simulink model "BAS_MPC_TV"  (R2018b)
settings: Solver=VariableStepAuto  StartTime=0.0  StopTime=10.0  RelTol=1e-3
values from neighbouring files (symbols this model uses):
  a = 1    [adaptive_mpc_tv.mat]
  b = 0.5    [adaptive_mpc_tv.mat]
  Izz = 100    [adaptive_mpc_tv.mat]
  M = 300    [adaptive_mpc_tv.mat]
  Rt = 0.226    [adaptive_mpc_tv.mat]
  track = 1.2    [adaptive_mpc_tv.mat]
  Ts = 0.02    [adaptive_mpc_tv.mat]
(part 1 of 2)
settings Model: Creator=littune  LastModifiedBy=littune

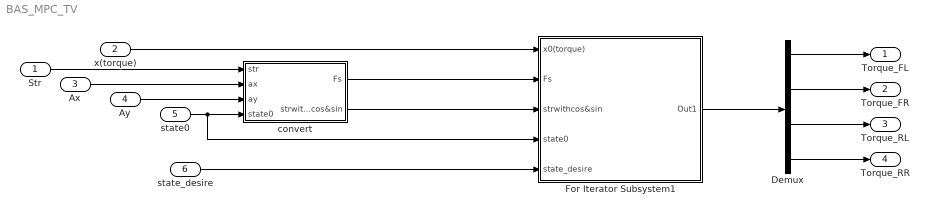
== system BAS_MPC_TV ==
  Str : Inport
  x(torque) : Inport  Port=2
  Ax : Inport  Port=3
  Ay : Inport  Port=4
  state0 : Inport  Port=5
  state_desire : Inport  Port=6
  Demux : Demux
  For Iterator Subsystem1 : Subsystem  TreatAsAtomicUnit=on
  convert : Subsystem
  Torque_FL : Outport
  Torque_FR : Outport  Port=2
  Torque_RL : Outport  Port=3
  Torque_RR : Outport  Port=4
  wires:
  convert/1(Fs) -> For Iterator Subsystem1/2(Fs)
  convert/2(strwithcos&sin) -> For Iterator Subsystem1/3(strwithcos&sin)
  Str/1 -> convert/1(str)
  x(torque)/1 -> For Iterator Subsystem1/1(x0(torque))
  Ax/1 -> convert/2(ax)
  Ay/1 -> convert/3(ay)
  state0/1 -> For Iterator Subsystem1/4(state0), convert/4(state0)
  state_desire/1 -> For Iterator Subsystem1/5(state_desire)
  For Iterator Subsystem1/1(Out1) -> Demux/1
  Demux/1 -> Torque_FL/1
  Demux/2 -> Torque_FR/1
  Demux/3 -> Torque_RL/1
  Demux/4 -> Torque_RR/1

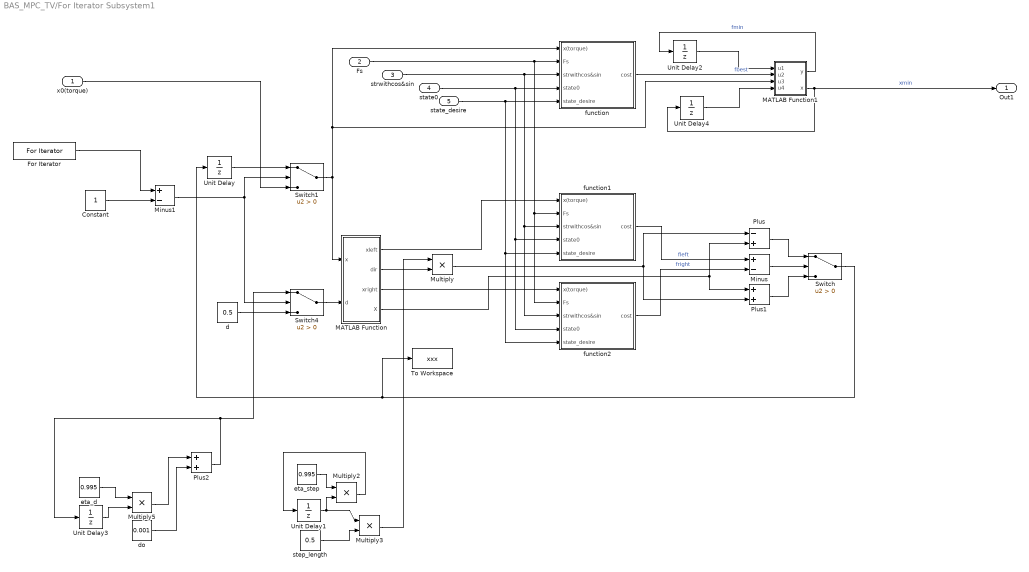
== system BAS_MPC_TV/For Iterator Subsystem1 ==
  x0(torque) : Inport
  Fs : Inport  Port=2
  strwithcos&sin : Inport  Port=3
  state0 : Inport  Port=4
  state_desire : Inport  Port=5
  Constant : Constant
  For Iterator : ForIterator  ResetStates=reset  IterationLimit=200
  MATLAB Function : MATLAB Function  TreatAsAtomicUnit=on
  MATLAB Function1 : MATLAB Function  TreatAsAtomicUnit=on
  Minus : Sum  Inputs=+-
  Minus1 : Sum  Inputs=+-
  Multiply{,2..3,5} (4 alike) : Product
  Plus : Sum  Inputs=-+
  Plus1 : Sum
  Plus2 : Sum
  Switch : Switch  Criteria=u2 > Threshold
  Switch1 : Switch  Criteria=u2 > Threshold
  Switch4 : Switch  Criteria=u2 > Threshold
  To Workspace : ToWorkspace  VariableName=xxx  SaveFormat=Timeseries  SampleTime=-1
  Unit Delay : UnitDelay  SampleTime=-1
  Unit Delay1 : UnitDelay  InitialCondition=1  SampleTime=-1
  Unit Delay2 : UnitDelay  InitialCondition=inf  SampleTime=-1
  Unit Delay3 : UnitDelay  InitialCondition=0.5  SampleTime=-1
  Unit Delay4 : UnitDelay  SampleTime=-1
  d : Constant  Value=0.5
  do : Constant  Value=0.001
  eta_d : Constant  Value=0.995
  eta_step : Constant  Value=0.995
  function : Subsystem
  function1 : Subsystem
  function2 : Subsystem
  step_length : Constant  Value=0.5
  Out1 : Outport
  wires:
  MATLAB Function/1(xleft) -> function1/1(x(torque))
  function/1(cost) -> MATLAB Function1/2(u2)  "fbest"
  strwithcos&sin/1 -> function/3(strwithcos&sin), function2/3(strwithcos&sin), function1/3(strwithcos&sin)
  MATLAB Function/3(xright) -> function2/1(x(torque))
  state0/1 -> function/4(state0), function2/4(state0), function1/4(state0)
  state_desire/1 -> function/5(state_desire), function2/5(state_desire), function1/5(state_desire)
  Fs/1 -> function/2(Fs), function2/2(Fs), function1/2(Fs)
  function1/1(cost) -> Minus/1  "fleft"
  function2/1(cost) -> Minus/2  "fright"
  Minus/1 -> Switch/2
  MATLAB Function/2(dir) -> Multiply/2
  Multiply/1 -> Plus/1, Plus1/2
  MATLAB Function/4(X) -> Plus1/1, Plus/2
  Plus/1 -> Switch/1
  Plus1/1 -> Switch/3
  Switch/1 -> Unit Delay/1, To Workspace/1
  Unit Delay/1 -> Switch1/1
  Switch1/1 -> MATLAB Function/1(x), function/1(x(torque)), MATLAB Function1/3(u3)
  Constant/1 -> Minus1/2
  Minus1/1 -> Switch4/2, Switch1/2
  eta_step/1 -> Multiply2/1
  Multiply2/1 -> Unit Delay1/1
  Unit Delay1/1 -> Multiply3/1, Multiply2/2
  step_length/1 -> Multiply3/2
  Multiply3/1 -> Multiply/1
  For Iterator/1 -> Minus1/1
  Multiply5/1 -> Plus2/1
  do/1 -> Plus2/2
  Switch4/1 -> MATLAB Function/2(d)
  d/1 -> Switch4/3
  Plus2/1 -> Switch4/1, Unit Delay3/1
  Unit Delay3/1 -> Multiply5/2
  eta_d/1 -> Multiply5/1
  x0(torque)/1 -> Switch1/3
  Unit Delay2/1 -> MATLAB Function1/1(u1)
  MATLAB Function1/1(y) -> Unit Delay2/1  "fmin"
  Unit Delay4/1 -> MATLAB Function1/4(u4)
  MATLAB Function1/2(x) -> Unit Delay4/1, Out1/1  "xmin"

== system BAS_MPC_TV/convert ==
  str : Inport
  ax : Inport  Port=2
  ay : Inport  Port=3
  state0 : Inport  Port=4
  Cos : Trigonometry  Operator=cos
  Cos1 : Trigonometry  Operator=cos
  Demux : Demux  Outputs=3
  MATLAB Function : MATLAB Function  TreatAsAtomicUnit=on
  MATLAB Function1 : MATLAB Function  TreatAsAtomicUnit=on
  Multiply{,1..3} (4 alike) : Product
  Mux : Mux
  Mux1 : Mux  Inputs=5
  Sin : Trigonometry
  Sin1 : Trigonometry
  ratio : Gain  Gain=1/5
  Fs : Outport
  strwithcos&sin : Outport  Port=2
  wires:
  ratio/1 -> Cos/1, Sin/1, Cos1/1, Mux1/5, Sin1/1
  str/1 -> ratio/1
  MATLAB Function/2(Fzfr) -> Multiply1/1
  ax/1 -> MATLAB Function/1(ax)
  ay/1 -> MATLAB Function/2(ay)
  Mux/1 -> Fs/1  "Fs"
  Mux1/1 -> strwithcos&sin/1  "strwithcos&sin"
  MATLAB Function1/4(usrr) -> Multiply3/2
  Sin/1 -> Mux1/1
  Multiply2/1 -> Mux/3  "Fs_RL"
  Multiply3/1 -> Mux/4  "Fs_RR"
  Multiply1/1 -> Mux/2  "Fs_FR"
  Multiply/1 -> Mux/1  "Fs_FL"
  MATLAB Function/4(Fzrr) -> Multiply3/1
  MATLAB Function/3(Fzrl) -> Multiply2/1
  Cos/1 -> Mux1/2
  Demux/2 -> MATLAB Function1/2(Vy0)
  state0/1 -> Demux/1
  MATLAB Function1/2(usfr) -> Multiply1/2
  Demux/3 -> MATLAB Function1/3(yawrate0)
  MATLAB Function1/3(usrl) -> Multiply2/2
  Cos1/1 -> Mux1/4
  Sin1/1 -> Mux1/3
  MATLAB Function1/1(usfl) -> Multiply/2
  Demux/1 -> MATLAB Function1/1(Vx0)
  MATLAB Function/1(Fzfl) -> Multiply/1

== system BAS_MPC_TV/For Iterator Subsystem1/function ==
  x(torque) : Inport
  Fs : Inport  Port=2
  strwithcos&sin : Inport  Port=3
  state0 : Inport  Port=4
  state_desire : Inport  Port=5
  10layer_model : Subsystem
  Gain : Gain  Gain=1/Rt
  Limitation : Subsystem
  SumFx : Subsystem
  SumFx1 : Subsystem
  cost : Outport
  wires:
  Gain/1 -> SumFx1/3(Ft), SumFx/3(Ft)
  state_desire/1 -> 10layer_model/4(state_desire)
  state0/1 -> 10layer_model/3(state0)
  strwithcos&sin/1 -> SumFx1/1(Strwithcos&sin), SumFx/1(Strwithcos&sin)
  x(torque)/1 -> Gain/1
  SumFx/1(Fx) -> 10layer_model/1(Fx)
  SumFx1/1(Fy) -> 10layer_model/2(Fy)
  Fs/1 -> SumFx/2(Fs), SumFx1/2(Fs)
  10layer_model/1(Fun) -> cost/1

== system BAS_MPC_TV/For Iterator Subsystem1/function1 ==
  x(torque) : Inport
  Fs : Inport  Port=2
  strwithcos&sin : Inport  Port=3
  state0 : Inport  Port=4
  state_desire : Inport  Port=5
  10layer_model : Subsystem
  Gain : Gain  Gain=1/Rt
  SumFx : Subsystem
  SumFx1 : Subsystem
  cost : Outport
  wires:
  Gain/1 -> SumFx1/3(Ft), SumFx/3(Ft)
  state_desire/1 -> 10layer_model/4(state_desire)
  state0/1 -> 10layer_model/3(state0)
  strwithcos&sin/1 -> SumFx1/1(Strwithcos&sin), SumFx/1(Strwithcos&sin)
  x(torque)/1 -> Gain/1
  SumFx/1(Fx) -> 10layer_model/1(Fx)
  SumFx1/1(Fy) -> 10layer_model/2(Fy)
  Fs/1 -> SumFx/2(Fs), SumFx1/2(Fs)
  10layer_model/1(Fun) -> cost/1

== system BAS_MPC_TV/For Iterator Subsystem1/function2 ==
  x(torque) : Inport
  Fs : Inport  Port=2
  strwithcos&sin : Inport  Port=3
  state0 : Inport  Port=4
  state_desire : Inport  Port=5
  10layer_model : Subsystem
  Gain : Gain  Gain=1/Rt
  SumFx : Subsystem
  SumFx1 : Subsystem
  cost : Outport
  wires:
  Gain/1 -> SumFx1/3(Ft), SumFx/3(Ft)
  state_desire/1 -> 10layer_model/4(state_desire)
  state0/1 -> 10layer_model/3(state0)
  strwithcos&sin/1 -> SumFx1/1(Strwithcos&sin), SumFx/1(Strwithcos&sin)
  x(torque)/1 -> Gain/1
  SumFx/1(Fx) -> 10layer_model/1(Fx)
  SumFx1/1(Fy) -> 10layer_model/2(Fy)
  Fs/1 -> SumFx/2(Fs), SumFx1/2(Fs)
  10layer_model/1(Fun) -> cost/1

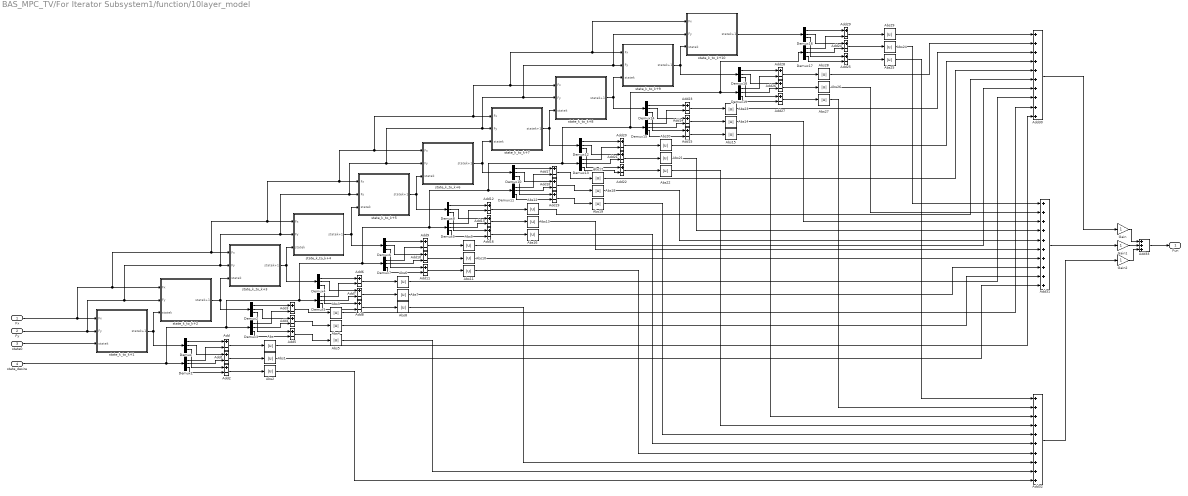
== system BAS_MPC_TV/For Iterator Subsystem1/function/10layer_model ==
  Fx : Inport
  Fy : Inport  Port=2
  state0 : Inport  Port=3
  state_desire : Inport  Port=4
  Abs{,1..29} (30 alike) : Abs
  Add{,1..29} (30 alike) : Sum  Inputs=+-
  Add30 : Sum  Inputs=10
  Add31 : Sum  Inputs=10
  Add32 : Sum  Inputs=10
  Add33 : Sum  Inputs=3
  Demux{,1..19} (20 alike) : Demux  Outputs=3
  Gain : Gain
  Gain1 : Gain
  Gain2 : Gain
  state_k_to_k+1 : Subsystem
  state_k_to_k+10 : Subsystem
  state_k_to_k+2 : Subsystem
  state_k_to_k+3 : Subsystem
  state_k_to_k+4 : Subsystem
  state_k_to_k+5 : Subsystem
  state_k_to_k+6 : Subsystem
  state_k_to_k+7 : Subsystem
  state_k_to_k+8 : Subsystem
  state_k_to_k+9 : Subsystem
  Fun : Outport
  wires:
  state_k_to_k+1/1(statek+1) -> state_k_to_k+2/3(statek), Demux/1
  state0/1 -> state_k_to_k+1/3(statek)
  Fx/1 -> state_k_to_k+10/1(Fx), state_k_to_k+9/1(Fx), state_k_to_k+8/1(Fx), state_k_to_k+7/1(Fx), state_k_to_k+6/1(Fx), state_k_to_k+5/1(Fx), state_k_to_k+4/1(Fx), state_k_to_k+3/1(Fx), state_k_to_k+2/1(Fx), state_k_to_k+1/1(Fx)
  Fy/1 -> state_k_to_k+10/2(Fy), state_k_to_k+9/2(Fy), state_k_to_k+8/2(Fy), state_k_to_k+7/2(Fy), state_k_to_k+6/2(Fy), state_k_to_k+5/2(Fy), state_k_to_k+4/2(Fy), state_k_to_k+3/2(Fy), state_k_to_k+2/2(Fy), state_k_to_k+1/2(Fy)
  Demux/1 -> Add/1
  Demux1/1 -> Add/2
  Demux/2 -> Add1/1
  Demux1/2 -> Add1/2
  Demux/3 -> Add2/1
  Demux1/3 -> Add2/2
  Add/1 -> Abs/1
  Add1/1 -> Abs1/1
  Add2/1 -> Abs2/1
  Demux2/1 -> Add3/1
  Demux2/3 -> Add5/1
  Demux3/3 -> Add5/2
  Demux2/2 -> Add4/1
  Demux3/1 -> Add3/2
  Add4/1 -> Abs4/1
  Add3/1 -> Abs3/1
  Add5/1 -> Abs5/1
  state_k_to_k+2/1(statek+1) -> Demux2/1, state_k_to_k+3/3(statek)
  Demux3/2 -> Add4/2
  Demux4/1 -> Add6/1
  Demux4/3 -> Add8/1
  Demux5/3 -> Add8/2
  Demux5/2 -> Add7/2
  Add11/1 -> Abs11/1
  Demux7/2 -> Add10/2
  Demux6/2 -> Add10/1
  Demux7/3 -> Add11/2
  Demux4/2 -> Add7/1
  Demux5/1 -> Add6/2
  Add10/1 -> Abs10/1
  Add9/1 -> Abs9/1
  Demux7/1 -> Add9/2
  Add6/1 -> Abs6/1
  Add8/1 -> Abs8/1
  Demux6/1 -> Add9/1
  Demux6/3 -> Add11/1
  Add7/1 -> Abs7/1
  state_k_to_k+4/1(statek+1) -> Demux6/1, state_k_to_k+5/3(statek)
  state_k_to_k+3/1(statek+1) -> Demux4/1, state_k_to_k+4/3(statek)
  state_k_to_k+7/1(statek+1) -> Demux12/1, state_k_to_k+8/3(statek)
  state_k_to_k+8/1(statek+1) -> Demux14/1, state_k_to_k+9/3(statek)
  Demux8/1 -> Add12/1
  Demux8/3 -> Add16/1
  Demux9/3 -> Add16/2
  Demux9/2 -> Add13/2
  Add19/1 -> Abs19/1
  Demux11/2 -> Add18/2
  Demux10/2 -> Add18/1
  Demux11/3 -> Add19/2
  Demux8/2 -> Add13/1
  Demux9/1 -> Add12/2
  Add18/1 -> Abs18/1
  Demux10/1 -> Add17/1
  Demux10/3 -> Add19/1
  Add12/1 -> Abs12/1
  Add21/1 -> Abs21/1
  Demux14/3 -> Add15/1
  Add16/1 -> Abs16/1
  Add20/1 -> Abs20/1
  Add17/1 -> Abs17/1
  Add22/1 -> Abs22/1
  Add23/1 -> Abs23/1
  Demux15/1 -> Add23/2
  Add14/1 -> Abs14/1
  Demux13/1 -> Add20/2
  Demux15/3 -> Add15/2
  Demux12/2 -> Add21/1
  Demux15/2 -> Add14/2
  Add15/1 -> Abs15/1
  Demux14/1 -> Add23/1
  Demux13/3 -> Add22/2
  Demux12/3 -> Add22/1
  Demux11/1 -> Add17/2
  Demux13/2 -> Add21/2
  Demux14/2 -> Add14/1
  Add13/1 -> Abs13/1
  state_k_to_k+6/1(statek+1) -> Demux10/1, state_k_to_k+7/3(statek)
  state_k_to_k+5/1(statek+1) -> Demux8/1, state_k_to_k+6/3(statek)
  Demux12/1 -> Add20/1
  Demux16/2 -> Add24/1
  state_k_to_k+10/1(statek+1) -> Demux16/1
  Add25/1 -> Abs25/1
  Demux17/3 -> Add25/2
  Add24/1 -> Abs24/1
  Demux16/1 -> Add29/1
  Demux17/2 -> Add24/2
  Demux16/3 -> Add25/1
  Demux17/1 -> Add29/2
  Add29/1 -> Abs29/1
  state_desire/1 -> Demux17/1, Demux19/1, Demux15/1, Demux13/1, Demux11/1, Demux9/1, Demux7/1, Demux5/1, Demux3/1, Demux1/1
  Add28/1 -> Abs28/1
  Demux19/2 -> Add26/2
  Demux19/1 -> Add28/2
  Demux18/1 -> Add28/1
  Demux18/3 -> Add27/1
  state_k_to_k+9/1(statek+1) -> Demux18/1, state_k_to_k+10/3(statek)
  Demux19/3 -> Add27/2
  Add27/1 -> Abs27/1
  Add26/1 -> Abs26/1
  Demux18/2 -> Add26/1
  Abs29/1 -> Add30/1
  Abs28/1 -> Add30/2
  Abs23/1 -> Add30/3
  Abs20/1 -> Add30/4
  Abs17/1 -> Add30/5
  Abs12/1 -> Add30/6
  Abs9/1 -> Add30/7
  Abs6/1 -> Add30/8
  Abs3/1 -> Add30/9
  Abs/1 -> Add30/10
  Add30/1 -> Gain/1
  Add31/1 -> Gain1/1
  Abs4/1 -> Add31/9
  Abs10/1 -> Add31/7
  Abs7/1 -> Add31/8
  Abs14/1 -> Add31/3
  Abs18/1 -> Add31/5
  Abs1/1 -> Add31/10
  Abs26/1 -> Add31/2
  Abs24/1 -> Add31/1
  Abs13/1 -> Add31/6
  Abs21/1 -> Add31/4
  Add32/1 -> Gain2/1
  Abs5/1 -> Add32/9
  Abs11/1 -> Add32/7
  Abs8/1 -> Add32/8
  Abs15/1 -> Add32/3
  Abs19/1 -> Add32/5
  Abs2/1 -> Add32/10
  Abs27/1 -> Add32/2
  Abs25/1 -> Add32/1
  Abs16/1 -> Add32/6
  Abs22/1 -> Add32/4
  Gain/1 -> Add33/1
  Gain1/1 -> Add33/2
  Gain2/1 -> Add33/3
  Add33/1 -> Fun/1

== system BAS_MPC_TV/For Iterator Subsystem1/function/Limitation ==
  Tire_limit : Inport
  In2 : Inport  Port=2
  MATLAB Function : MATLAB Function  TreatAsAtomicUnit=on
  Out1 : Outport

== system BAS_MPC_TV/For Iterator Subsystem1/function/SumFx ==
  Strwithcos&sin : Inport
  Fs : Inport  Port=2
  Ft : Inport  Port=3
  Add2 : Sum  Inputs=-+
  Add3 : Sum  Inputs=-+
  Demux : Demux
  Demux1 : Demux  Outputs=5
  Demux2 : Demux
  Multiply{1..4} (4 alike) : Product
  Mux : Mux
  Terminator : Terminator
  Terminator1 : Terminator
  Terminator2 : Terminator
  Fx : Outport
  wires:
  Demux/1 -> Multiply1/1  "Ft_FL"
  Demux/2 -> Multiply3/1  "Ft_FR"
  Demux/3 -> Mux/3  "Ft_RL"
  Demux/4 -> Mux/4  "Ft_RR"
  Demux1/1 -> Multiply2/2  "left sin"
  Demux1/2 -> Multiply1/2  "left cos"
  Demux1/3 -> Multiply4/2  "right sin"
  Demux1/4 -> Multiply3/2  "right cos"
  Ft/1 -> Demux/1
  Demux1/5 -> Terminator2/1  "str"
  Strwithcos&sin/1 -> Demux1/1
  Fs/1 -> Demux2/1
  Demux2/1 -> Multiply2/1  "Fs_FL"
  Demux2/2 -> Multiply4/1  "Fs_FR"
  Demux2/3 -> Terminator/1  "Fs_RL"
  Demux2/4 -> Terminator1/1  "Fs_RR"
  Multiply2/1 -> Add2/1
  Multiply1/1 -> Add2/2
  Add2/1 -> Mux/1  "Fx_FL"
  Multiply4/1 -> Add3/1
  Multiply3/1 -> Add3/2
  Add3/1 -> Mux/2  "Fx_FR"
  Mux/1 -> Fx/1

== system BAS_MPC_TV/For Iterator Subsystem1/function/SumFx1 ==
  Strwithcos&sin : Inport
  Fs : Inport  Port=2
  Ft : Inport  Port=3
  Add2 : Sum
  Add3 : Sum
  Demux : Demux
  Demux1 : Demux  Outputs=5
  Demux2 : Demux
  Multiply{1..4} (4 alike) : Product
  Mux : Mux
  Terminator1 : Terminator
  Terminator2 : Terminator
  Terminator3 : Terminator
  Fy : Outport
  wires:
  Demux/1 -> Multiply1/1  "Ft_FL"
  Demux/2 -> Multiply3/1  "Ft_FR"
  Demux/3 -> Terminator1/1  "Ft_RL"
  Demux/4 -> Terminator3/1  "Ft_RR"
  Demux1/1 -> Multiply1/2  "left sin"
  Demux1/2 -> Multiply2/2  "left cos"
  Demux1/3 -> Multiply3/2  "right sin"
  Demux1/4 -> Multiply4/2  "right cos"
  Ft/1 -> Demux/1
  Demux1/5 -> Terminator2/1  "str"
  Strwithcos&sin/1 -> Demux1/1
  Fs/1 -> Demux2/1
  Demux2/1 -> Multiply2/1  "Fs_FL"
  Demux2/2 -> Multiply4/1  "Fs_FR"
  Demux2/3 -> Mux/3  "Fs_RL"
  Demux2/4 -> Mux/4  "Fs_RR"
  Multiply2/1 -> Add2/1
  Multiply1/1 -> Add2/2
  Add2/1 -> Mux/1  "Fy_FL"
  Multiply4/1 -> Add3/1
  Multiply3/1 -> Add3/2
  Add3/1 -> Mux/2  "Fy_FR"
  Mux/1 -> Fy/1

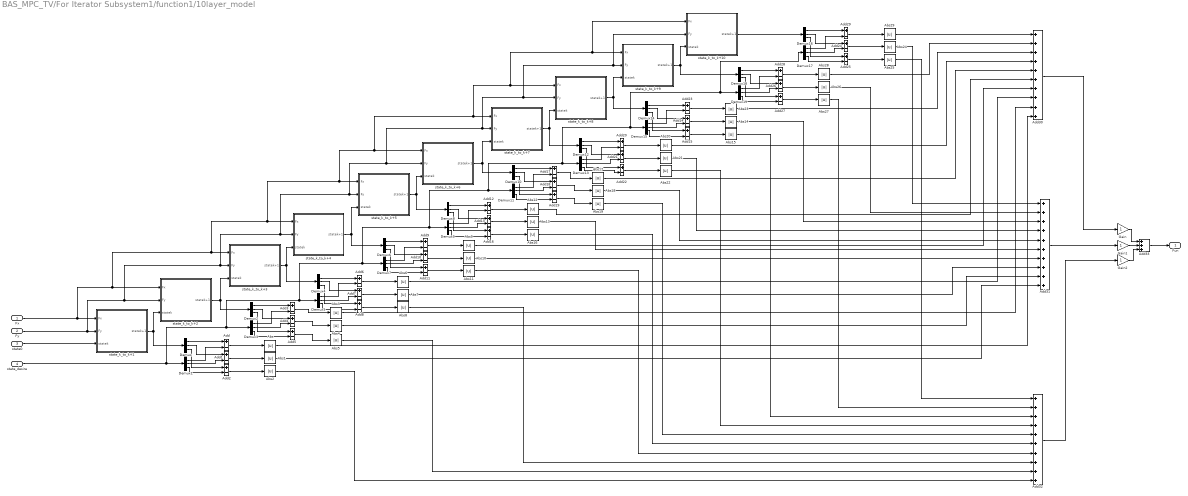
== system BAS_MPC_TV/For Iterator Subsystem1/function1/10layer_model ==
  Fx : Inport
  Fy : Inport  Port=2
  state0 : Inport  Port=3
  state_desire : Inport  Port=4
  Abs{,1..29} (30 alike) : Abs
  Add{,1..29} (30 alike) : Sum  Inputs=+-
  Add30 : Sum  Inputs=10
  Add31 : Sum  Inputs=10
  Add32 : Sum  Inputs=10
  Add33 : Sum  Inputs=3
  Demux{,1..19} (20 alike) : Demux  Outputs=3
  Gain : Gain
  Gain1 : Gain
  Gain2 : Gain
  state_k_to_k+1 : Subsystem
  state_k_to_k+10 : Subsystem
  state_k_to_k+2 : Subsystem
  state_k_to_k+3 : Subsystem
  state_k_to_k+4 : Subsystem
  state_k_to_k+5 : Subsystem
  state_k_to_k+6 : Subsystem
  state_k_to_k+7 : Subsystem
  state_k_to_k+8 : Subsystem
  state_k_to_k+9 : Subsystem
  Fun : Outport
  wires:
  state_k_to_k+1/1(statek+1) -> state_k_to_k+2/3(statek), Demux/1
  state0/1 -> state_k_to_k+1/3(statek)
  Fx/1 -> state_k_to_k+10/1(Fx), state_k_to_k+9/1(Fx), state_k_to_k+8/1(Fx), state_k_to_k+7/1(Fx), state_k_to_k+6/1(Fx), state_k_to_k+5/1(Fx), state_k_to_k+4/1(Fx), state_k_to_k+3/1(Fx), state_k_to_k+2/1(Fx), state_k_to_k+1/1(Fx)
  Fy/1 -> state_k_to_k+10/2(Fy), state_k_to_k+9/2(Fy), state_k_to_k+8/2(Fy), state_k_to_k+7/2(Fy), state_k_to_k+6/2(Fy), state_k_to_k+5/2(Fy), state_k_to_k+4/2(Fy), state_k_to_k+3/2(Fy), state_k_to_k+2/2(Fy), state_k_to_k+1/2(Fy)
  Demux/1 -> Add/1
  Demux1/1 -> Add/2
  Demux/2 -> Add1/1
  Demux1/2 -> Add1/2
  Demux/3 -> Add2/1
  Demux1/3 -> Add2/2
  Add/1 -> Abs/1
  Add1/1 -> Abs1/1
  Add2/1 -> Abs2/1
  Demux2/1 -> Add3/1
  Demux2/3 -> Add5/1
  Demux3/3 -> Add5/2
  Demux2/2 -> Add4/1
  Demux3/1 -> Add3/2
  Add4/1 -> Abs4/1
  Add3/1 -> Abs3/1
  Add5/1 -> Abs5/1
  state_k_to_k+2/1(statek+1) -> Demux2/1, state_k_to_k+3/3(statek)
  Demux3/2 -> Add4/2
  Demux4/1 -> Add6/1
  Demux4/3 -> Add8/1
  Demux5/3 -> Add8/2
  Demux5/2 -> Add7/2
  Add11/1 -> Abs11/1
  Demux7/2 -> Add10/2
  Demux6/2 -> Add10/1
  Demux7/3 -> Add11/2
  Demux4/2 -> Add7/1
  Demux5/1 -> Add6/2
  Add10/1 -> Abs10/1
  Add9/1 -> Abs9/1
  Demux7/1 -> Add9/2
  Add6/1 -> Abs6/1
  Add8/1 -> Abs8/1
  Demux6/1 -> Add9/1
  Demux6/3 -> Add11/1
  Add7/1 -> Abs7/1
  state_k_to_k+4/1(statek+1) -> Demux6/1, state_k_to_k+5/3(statek)
  state_k_to_k+3/1(statek+1) -> Demux4/1, state_k_to_k+4/3(statek)
  state_k_to_k+7/1(statek+1) -> Demux12/1, state_k_to_k+8/3(statek)
  state_k_to_k+8/1(statek+1) -> Demux14/1, state_k_to_k+9/3(statek)
  Demux8/1 -> Add12/1
  Demux8/3 -> Add16/1
  Demux9/3 -> Add16/2
  Demux9/2 -> Add13/2
  Add19/1 -> Abs19/1
  Demux11/2 -> Add18/2
  Demux10/2 -> Add18/1
  Demux11/3 -> Add19/2
  Demux8/2 -> Add13/1
  Demux9/1 -> Add12/2
  Add18/1 -> Abs18/1
  Demux10/1 -> Add17/1
  Demux10/3 -> Add19/1
  Add12/1 -> Abs12/1
  Add21/1 -> Abs21/1
  Demux14/3 -> Add15/1
  Add16/1 -> Abs16/1
  Add20/1 -> Abs20/1
  Add17/1 -> Abs17/1
  Add22/1 -> Abs22/1
  Add23/1 -> Abs23/1
  Demux15/1 -> Add23/2
  Add14/1 -> Abs14/1
  Demux13/1 -> Add20/2
  Demux15/3 -> Add15/2
  Demux12/2 -> Add21/1
  Demux15/2 -> Add14/2
  Add15/1 -> Abs15/1
  Demux14/1 -> Add23/1
  Demux13/3 -> Add22/2
  Demux12/3 -> Add22/1
  Demux11/1 -> Add17/2
  Demux13/2 -> Add21/2
  Demux14/2 -> Add14/1
  Add13/1 -> Abs13/1
  state_k_to_k+6/1(statek+1) -> Demux10/1, state_k_to_k+7/3(statek)
  state_k_to_k+5/1(statek+1) -> Demux8/1, state_k_to_k+6/3(statek)
  Demux12/1 -> Add20/1
  Demux16/2 -> Add24/1
  state_k_to_k+10/1(statek+1) -> Demux16/1
  Add25/1 -> Abs25/1
  Demux17/3 -> Add25/2
  Add24/1 -> Abs24/1
  Demux16/1 -> Add29/1
  Demux17/2 -> Add24/2
  Demux16/3 -> Add25/1
  Demux17/1 -> Add29/2
  Add29/1 -> Abs29/1
  state_desire/1 -> Demux17/1, Demux19/1, Demux15/1, Demux13/1, Demux11/1, Demux9/1, Demux7/1, Demux5/1, Demux3/1, Demux1/1
  Add28/1 -> Abs28/1
  Demux19/2 -> Add26/2
  Demux19/1 -> Add28/2
  Demux18/1 -> Add28/1
  Demux18/3 -> Add27/1
  state_k_to_k+9/1(statek+1) -> Demux18/1, state_k_to_k+10/3(statek)
  Demux19/3 -> Add27/2
  Add27/1 -> Abs27/1
  Add26/1 -> Abs26/1
  Demux18/2 -> Add26/1
  Abs29/1 -> Add30/1
  Abs28/1 -> Add30/2
  Abs23/1 -> Add30/3
  Abs20/1 -> Add30/4
  Abs17/1 -> Add30/5
  Abs12/1 -> Add30/6
  Abs9/1 -> Add30/7
  Abs6/1 -> Add30/8
  Abs3/1 -> Add30/9
  Abs/1 -> Add30/10
  Add30/1 -> Gain/1
  Add31/1 -> Gain1/1
  Abs4/1 -> Add31/9
  Abs10/1 -> Add31/7
  Abs7/1 -> Add31/8
  Abs14/1 -> Add31/3
  Abs18/1 -> Add31/5
  Abs1/1 -> Add31/10
  Abs26/1 -> Add31/2
  Abs24/1 -> Add31/1
  Abs13/1 -> Add31/6
  Abs21/1 -> Add31/4
  Add32/1 -> Gain2/1
  Abs5/1 -> Add32/9
  Abs11/1 -> Add32/7
  Abs8/1 -> Add32/8
  Abs15/1 -> Add32/3
  Abs19/1 -> Add32/5
  Abs2/1 -> Add32/10
  Abs27/1 -> Add32/2
  Abs25/1 -> Add32/1
  Abs16/1 -> Add32/6
  Abs22/1 -> Add32/4
  Gain/1 -> Add33/1
  Gain1/1 -> Add33/2
  Gain2/1 -> Add33/3
  Add33/1 -> Fun/1

== system BAS_MPC_TV/For Iterator Subsystem1/function1/SumFx ==
  Strwithcos&sin : Inport
  Fs : Inport  Port=2
  Ft : Inport  Port=3
  Add2 : Sum  Inputs=-+
  Add3 : Sum  Inputs=-+
  Demux : Demux
  Demux1 : Demux  Outputs=5
  Demux2 : Demux
  Multiply{1..4} (4 alike) : Product
  Mux : Mux
  Terminator : Terminator
  Terminator1 : Terminator
  Terminator2 : Terminator
  Fx : Outport
  wires:
  Demux/1 -> Multiply1/1  "Ft_FL"
  Demux/2 -> Multiply3/1  "Ft_FR"
  Demux/3 -> Mux/3  "Ft_RL"
  Demux/4 -> Mux/4  "Ft_RR"
  Demux1/1 -> Multiply2/2  "left sin"
  Demux1/2 -> Multiply1/2  "left cos"
  Demux1/3 -> Multiply4/2  "right sin"
  Demux1/4 -> Multiply3/2  "right cos"
  Ft/1 -> Demux/1
  Demux1/5 -> Terminator2/1  "str"
  Strwithcos&sin/1 -> Demux1/1
  Fs/1 -> Demux2/1
  Demux2/1 -> Multiply2/1  "Fs_FL"
  Demux2/2 -> Multiply4/1  "Fs_FR"
  Demux2/3 -> Terminator/1  "Fs_RL"
  Demux2/4 -> Terminator1/1  "Fs_RR"
  Multiply2/1 -> Add2/1
  Multiply1/1 -> Add2/2
  Add2/1 -> Mux/1  "Fx_FL"
  Multiply4/1 -> Add3/1
  Multiply3/1 -> Add3/2
  Add3/1 -> Mux/2  "Fx_FR"
  Mux/1 -> Fx/1

== system BAS_MPC_TV/For Iterator Subsystem1/function1/SumFx1 ==
  Strwithcos&sin : Inport
  Fs : Inport  Port=2
  Ft : Inport  Port=3
  Add2 : Sum
  Add3 : Sum
  Demux : Demux
  Demux1 : Demux  Outputs=5
  Demux2 : Demux
  Multiply{1..4} (4 alike) : Product
  Mux : Mux
  Terminator1 : Terminator
  Terminator2 : Terminator
  Terminator3 : Terminator
  Fy : Outport
  wires:
  Demux/1 -> Multiply1/1  "Ft_FL"
  Demux/2 -> Multiply3/1  "Ft_FR"
  Demux/3 -> Terminator1/1  "Ft_RL"
  Demux/4 -> Terminator3/1  "Ft_RR"
  Demux1/1 -> Multiply1/2  "left sin"
  Demux1/2 -> Multiply2/2  "left cos"
  Demux1/3 -> Multiply3/2  "right sin"
  Demux1/4 -> Multiply4/2  "right cos"
  Ft/1 -> Demux/1
  Demux1/5 -> Terminator2/1  "str"
  Strwithcos&sin/1 -> Demux1/1
  Fs/1 -> Demux2/1
  Demux2/1 -> Multiply2/1  "Fs_FL"
  Demux2/2 -> Multiply4/1  "Fs_FR"
  Demux2/3 -> Mux/3  "Fs_RL"
  Demux2/4 -> Mux/4  "Fs_RR"
  Multiply2/1 -> Add2/1
  Multiply1/1 -> Add2/2
  Add2/1 -> Mux/1  "Fy_FL"
  Multiply4/1 -> Add3/1
  Multiply3/1 -> Add3/2
  Add3/1 -> Mux/2  "Fy_FR"
  Mux/1 -> Fy/1

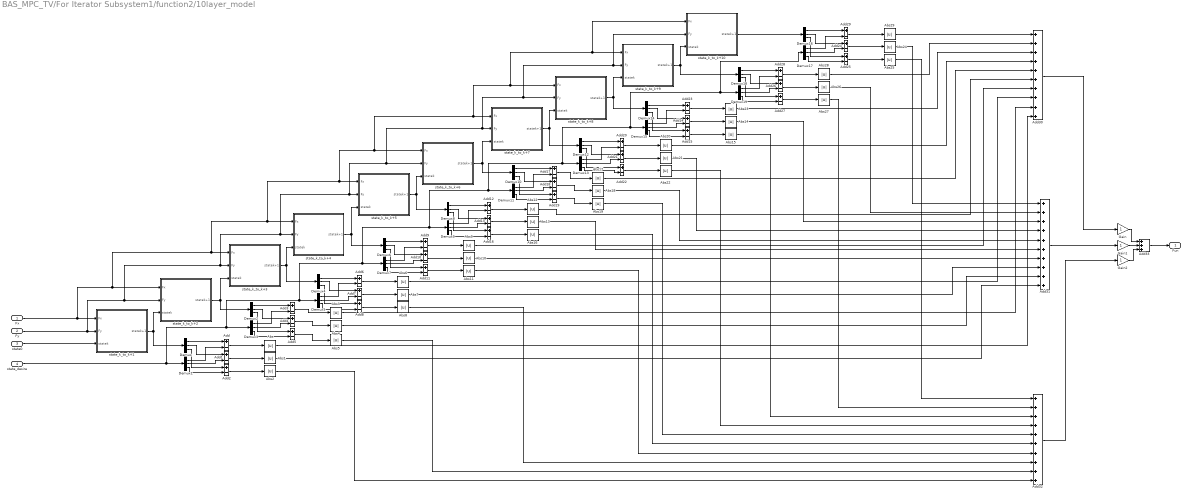
== system BAS_MPC_TV/For Iterator Subsystem1/function2/10layer_model ==
  Fx : Inport
  Fy : Inport  Port=2
  state0 : Inport  Port=3
  state_desire : Inport  Port=4
  Abs{,1..29} (30 alike) : Abs
  Add{,1..29} (30 alike) : Sum  Inputs=+-
  Add30 : Sum  Inputs=10
  Add31 : Sum  Inputs=10
  Add32 : Sum  Inputs=10
  Add33 : Sum  Inputs=3
  Demux{,1..19} (20 alike) : Demux  Outputs=3
  Gain : Gain
  Gain1 : Gain
  Gain2 : Gain
  state_k_to_k+1 : Subsystem
  state_k_to_k+10 : Subsystem
  state_k_to_k+2 : Subsystem
  state_k_to_k+3 : Subsystem
  state_k_to_k+4 : Subsystem
  state_k_to_k+5 : Subsystem
  state_k_to_k+6 : Subsystem
  state_k_to_k+7 : Subsystem
  state_k_to_k+8 : Subsystem
  state_k_to_k+9 : Subsystem
  Fun : Outport
  wires:
  state_k_to_k+1/1(statek+1) -> state_k_to_k+2/3(statek), Demux/1
  state0/1 -> state_k_to_k+1/3(statek)
  Fx/1 -> state_k_to_k+10/1(Fx), state_k_to_k+9/1(Fx), state_k_to_k+8/1(Fx), state_k_to_k+7/1(Fx), state_k_to_k+6/1(Fx), state_k_to_k+5/1(Fx), state_k_to_k+4/1(Fx), state_k_to_k+3/1(Fx), state_k_to_k+2/1(Fx), state_k_to_k+1/1(Fx)
  Fy/1 -> state_k_to_k+10/2(Fy), state_k_to_k+9/2(Fy), state_k_to_k+8/2(Fy), state_k_to_k+7/2(Fy), state_k_to_k+6/2(Fy), state_k_to_k+5/2(Fy), state_k_to_k+4/2(Fy), state_k_to_k+3/2(Fy), state_k_to_k+2/2(Fy), state_k_to_k+1/2(Fy)
  Demux/1 -> Add/1
  Demux1/1 -> Add/2
  Demux/2 -> Add1/1
  Demux1/2 -> Add1/2
  Demux/3 -> Add2/1
  Demux1/3 -> Add2/2
  Add/1 -> Abs/1
  Add1/1 -> Abs1/1
  Add2/1 -> Abs2/1
  Demux2/1 -> Add3/1
  Demux2/3 -> Add5/1
  Demux3/3 -> Add5/2
  Demux2/2 -> Add4/1
  Demux3/1 -> Add3/2
  Add4/1 -> Abs4/1
  Add3/1 -> Abs3/1
  Add5/1 -> Abs5/1
  state_k_to_k+2/1(statek+1) -> Demux2/1, state_k_to_k+3/3(statek)
  Demux3/2 -> Add4/2
  Demux4/1 -> Add6/1
  Demux4/3 -> Add8/1
  Demux5/3 -> Add8/2
  Demux5/2 -> Add7/2
  Add11/1 -> Abs11/1
  Demux7/2 -> Add10/2
  Demux6/2 -> Add10/1
  Demux7/3 -> Add11/2
  Demux4/2 -> Add7/1
  Demux5/1 -> Add6/2
  Add10/1 -> Abs10/1
  Add9/1 -> Abs9/1
  Demux7/1 -> Add9/2
  Add6/1 -> Abs6/1
  Add8/1 -> Abs8/1
  Demux6/1 -> Add9/1
  Demux6/3 -> Add11/1
  Add7/1 -> Abs7/1
  state_k_to_k+4/1(statek+1) -> Demux6/1, state_k_to_k+5/3(statek)
  state_k_to_k+3/1(statek+1) -> Demux4/1, state_k_to_k+4/3(statek)
  state_k_to_k+7/1(statek+1) -> Demux12/1, state_k_to_k+8/3(statek)
  state_k_to_k+8/1(statek+1) -> Demux14/1, state_k_to_k+9/3(statek)
  Demux8/1 -> Add12/1
  Demux8/3 -> Add16/1
  Demux9/3 -> Add16/2
  Demux9/2 -> Add13/2
  Add19/1 -> Abs19/1
  Demux11/2 -> Add18/2
  Demux10/2 -> Add18/1
  Demux11/3 -> Add19/2
  Demux8/2 -> Add13/1
  Demux9/1 -> Add12/2
  Add18/1 -> Abs18/1
  Demux10/1 -> Add17/1
  Demux10/3 -> Add19/1
  Add12/1 -> Abs12/1
  Add21/1 -> Abs21/1
  Demux14/3 -> Add15/1
  Add16/1 -> Abs16/1
  Add20/1 -> Abs20/1
  Add17/1 -> Abs17/1
  Add22/1 -> Abs22/1
  Add23/1 -> Abs23/1
  Demux15/1 -> Add23/2
  Add14/1 -> Abs14/1
  Demux13/1 -> Add20/2
  Demux15/3 -> Add15/2
  Demux12/2 -> Add21/1
  Demux15/2 -> Add14/2
  Add15/1 -> Abs15/1
  Demux14/1 -> Add23/1
  Demux13/3 -> Add22/2
  Demux12/3 -> Add22/1
  Demux11/1 -> Add17/2
  Demux13/2 -> Add21/2
  Demux14/2 -> Add14/1
  Add13/1 -> Abs13/1
  state_k_to_k+6/1(statek+1) -> Demux10/1, state_k_to_k+7/3(statek)
  state_k_to_k+5/1(statek+1) -> Demux8/1, state_k_to_k+6/3(statek)
  Demux12/1 -> Add20/1
  Demux16/2 -> Add24/1
  state_k_to_k+10/1(statek+1) -> Demux16/1
  Add25/1 -> Abs25/1
  Demux17/3 -> Add25/2
  Add24/1 -> Abs24/1
  Demux16/1 -> Add29/1
  Demux17/2 -> Add24/2
  Demux16/3 -> Add25/1
  Demux17/1 -> Add29/2
  Add29/1 -> Abs29/1
  state_desire/1 -> Demux17/1, Demux19/1, Demux15/1, Demux13/1, Demux11/1, Demux9/1, Demux7/1, Demux5/1, Demux3/1, Demux1/1
  Add28/1 -> Abs28/1
  Demux19/2 -> Add26/2
  Demux19/1 -> Add28/2
  Demux18/1 -> Add28/1
  Demux18/3 -> Add27/1
  state_k_to_k+9/1(statek+1) -> Demux18/1, state_k_to_k+10/3(statek)
  Demux19/3 -> Add27/2
  Add27/1 -> Abs27/1
  Add26/1 -> Abs26/1
  Demux18/2 -> Add26/1
  Abs29/1 -> Add30/1
  Abs28/1 -> Add30/2
  Abs23/1 -> Add30/3
  Abs20/1 -> Add30/4
  Abs17/1 -> Add30/5
  Abs12/1 -> Add30/6
  Abs9/1 -> Add30/7
  Abs6/1 -> Add30/8
  Abs3/1 -> Add30/9
  Abs/1 -> Add30/10
  Add30/1 -> Gain/1
  Add31/1 -> Gain1/1
  Abs4/1 -> Add31/9
  Abs10/1 -> Add31/7
  Abs7/1 -> Add31/8
  Abs14/1 -> Add31/3
  Abs18/1 -> Add31/5
  Abs1/1 -> Add31/10
  Abs26/1 -> Add31/2
  Abs24/1 -> Add31/1
  Abs13/1 -> Add31/6
  Abs21/1 -> Add31/4
  Add32/1 -> Gain2/1
  Abs5/1 -> Add32/9
  Abs11/1 -> Add32/7
  Abs8/1 -> Add32/8
  Abs15/1 -> Add32/3
  Abs19/1 -> Add32/5
  Abs2/1 -> Add32/10
  Abs27/1 -> Add32/2
  Abs25/1 -> Add32/1
  Abs16/1 -> Add32/6
  Abs22/1 -> Add32/4
  Gain/1 -> Add33/1
  Gain1/1 -> Add33/2
  Gain2/1 -> Add33/3
  Add33/1 -> Fun/1

== system BAS_MPC_TV/For Iterator Subsystem1/function2/SumFx ==
  Strwithcos&sin : Inport
  Fs : Inport  Port=2
  Ft : Inport  Port=3
  Add2 : Sum  Inputs=-+
  Add3 : Sum  Inputs=-+
  Demux : Demux
  Demux1 : Demux  Outputs=5
  Demux2 : Demux
  Multiply{1..4} (4 alike) : Product
  Mux : Mux
  Terminator : Terminator
  Terminator1 : Terminator
  Terminator2 : Terminator
  Fx : Outport
  wires:
  Demux/1 -> Multiply1/1  "Ft_FL"
  Demux/2 -> Multiply3/1  "Ft_FR"
  Demux/3 -> Mux/3  "Ft_RL"
  Demux/4 -> Mux/4  "Ft_RR"
  Demux1/1 -> Multiply2/2  "left sin"
  Demux1/2 -> Multiply1/2  "left cos"
  Demux1/3 -> Multiply4/2  "right sin"
  Demux1/4 -> Multiply3/2  "right cos"
  Ft/1 -> Demux/1
  Demux1/5 -> Terminator2/1  "str"
  Strwithcos&sin/1 -> Demux1/1
  Fs/1 -> Demux2/1
  Demux2/1 -> Multiply2/1  "Fs_FL"
  Demux2/2 -> Multiply4/1  "Fs_FR"
  Demux2/3 -> Terminator/1  "Fs_RL"
  Demux2/4 -> Terminator1/1  "Fs_RR"
  Multiply2/1 -> Add2/1
  Multiply1/1 -> Add2/2
  Add2/1 -> Mux/1  "Fx_FL"
  Multiply4/1 -> Add3/1
  Multiply3/1 -> Add3/2
  Add3/1 -> Mux/2  "Fx_FR"
  Mux/1 -> Fx/1

== system BAS_MPC_TV/For Iterator Subsystem1/function2/SumFx1 ==
  Strwithcos&sin : Inport
  Fs : Inport  Port=2
  Ft : Inport  Port=3
  Add2 : Sum
  Add3 : Sum
  Demux : Demux
  Demux1 : Demux  Outputs=5
  Demux2 : Demux
  Multiply{1..4} (4 alike) : Product
  Mux : Mux
  Terminator1 : Terminator
  Terminator2 : Terminator
  Terminator3 : Terminator
  Fy : Outport
  wires:
  Demux/1 -> Multiply1/1  "Ft_FL"
  Demux/2 -> Multiply3/1  "Ft_FR"
  Demux/3 -> Terminator1/1  "Ft_RL"
  Demux/4 -> Terminator3/1  "Ft_RR"
  Demux1/1 -> Multiply1/2  "left sin"
  Demux1/2 -> Multiply2/2  "left cos"
  Demux1/3 -> Multiply3/2  "right sin"
  Demux1/4 -> Multiply4/2  "right cos"
  Ft/1 -> Demux/1
  Demux1/5 -> Terminator2/1  "str"
  Strwithcos&sin/1 -> Demux1/1
  Fs/1 -> Demux2/1
  Demux2/1 -> Multiply2/1  "Fs_FL"
  Demux2/2 -> Multiply4/1  "Fs_FR"
  Demux2/3 -> Mux/3  "Fs_RL"
  Demux2/4 -> Mux/4  "Fs_RR"
  Multiply2/1 -> Add2/1
  Multiply1/1 -> Add2/2
  Add2/1 -> Mux/1  "Fy_FL"
  Multiply4/1 -> Add3/1
  Multiply3/1 -> Add3/2
  Add3/1 -> Mux/2  "Fy_FR"
  Mux/1 -> Fy/1

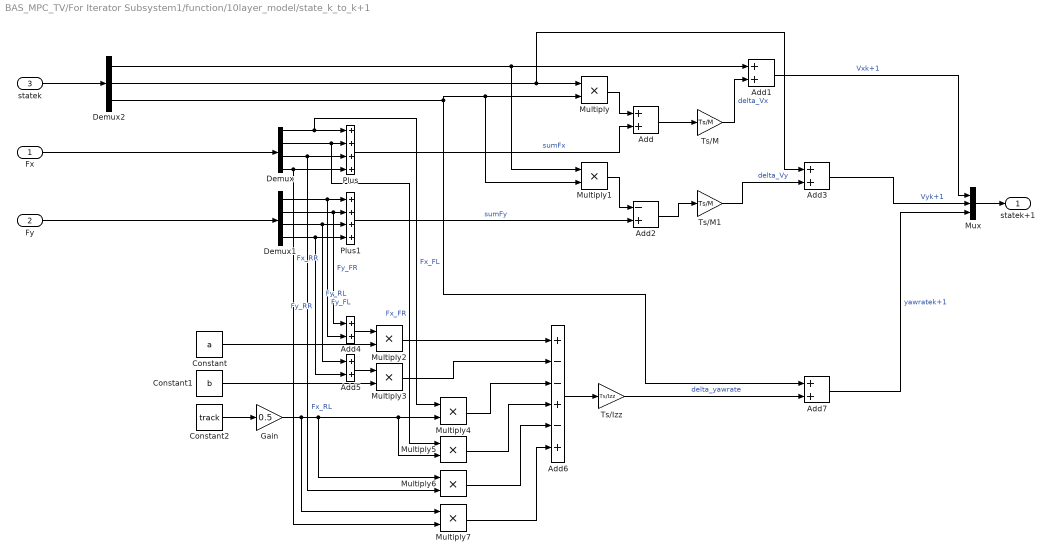
== system BAS_MPC_TV/For Iterator Subsystem1/function/10layer_model/state_k_to_k+1 ==
  Fx : Inport
  Fy : Inport  Port=2
  statek : Inport  Port=3
  Add{,1,3..5,7} (6 alike) : Sum
  Add2 : Sum  Inputs=-+
  Add6 : Sum  Inputs=+--+-+
  Constant : Constant  Value=a
  Constant1 : Constant  Value=b
  Constant2 : Constant  Value=track
  Demux : Demux
  Demux1 : Demux
  Demux2 : Demux  Outputs=3
  Gain : Gain  Gain=0.5
  Multiply{,1..7} (8 alike) : Product
  Mux : Mux  Inputs=3
  Plus : Sum  Inputs=4
  Plus1 : Sum  Inputs=4
  Ts/Izz : Gain  Gain=Ts/Izz
  Ts/M : Gain  Gain=Ts/M
  Ts/M1 : Gain  Gain=Ts/M
  statek+1 : Outport
  wires:
  Demux2/2 -> Add3/1, Multiply/1
  Demux2/3 -> Multiply1/2, Multiply/2, Add7/1
  Multiply/1 -> Add/1
  Add/1 -> Ts/M/1
  Ts/M/1 -> Add1/2  "delta_Vx"
  Demux2/1 -> Add1/1, Multiply1/1
  Add1/1 -> Mux/1  "Vxk+1"
  Fx/1 -> Demux/1
  Demux/1 -> Multiply4/1, Plus/1  "Fx_FL"
  Demux/2 -> Multiply5/1, Plus/2  "Fx_FR"
  Demux/3 -> Multiply6/2, Plus/3  "Fx_RL"
  Demux/4 -> Plus/4, Multiply7/2  "Fx_RR"
  Plus/1 -> Add/2  "sumFx"
  Demux1/3 -> Add5/1, Plus1/3  "Fy_RL"
  Demux1/2 -> Add4/1, Plus1/2  "Fy_FR"
  Demux1/1 -> Add4/2, Plus1/1  "Fy_FL"
  Demux1/4 -> Add5/2, Plus1/4  "Fy_RR"
  Fy/1 -> Demux1/1
  Plus1/1 -> Add2/2  "sumFy"
  Multiply1/1 -> Add2/1
  Add2/1 -> Ts/M1/1
  Ts/M1/1 -> Add3/2  "delta_Vy"
  Add3/1 -> Mux/2  "Vyk+1"
  Add4/1 -> Multiply2/1
  Constant/1 -> Multiply2/2
  Multiply2/1 -> Add6/1
  Multiply3/1 -> Add6/2
  Constant1/1 -> Multiply3/2
  Add5/1 -> Multiply3/1
  Constant2/1 -> Gain/1
  Gain/1 -> Multiply7/1, Multiply4/2, Multiply5/2, Multiply6/1
  Multiply4/1 -> Add6/3
  Multiply5/1 -> Add6/4
  Multiply6/1 -> Add6/5
  Multiply7/1 -> Add6/6
  Add6/1 -> Ts/Izz/1
  Ts/Izz/1 -> Add7/2  "delta_yawrate"
  Add7/1 -> Mux/3  "yawratek+1"
  statek/1 -> Demux2/1
  Mux/1 -> statek+1/1

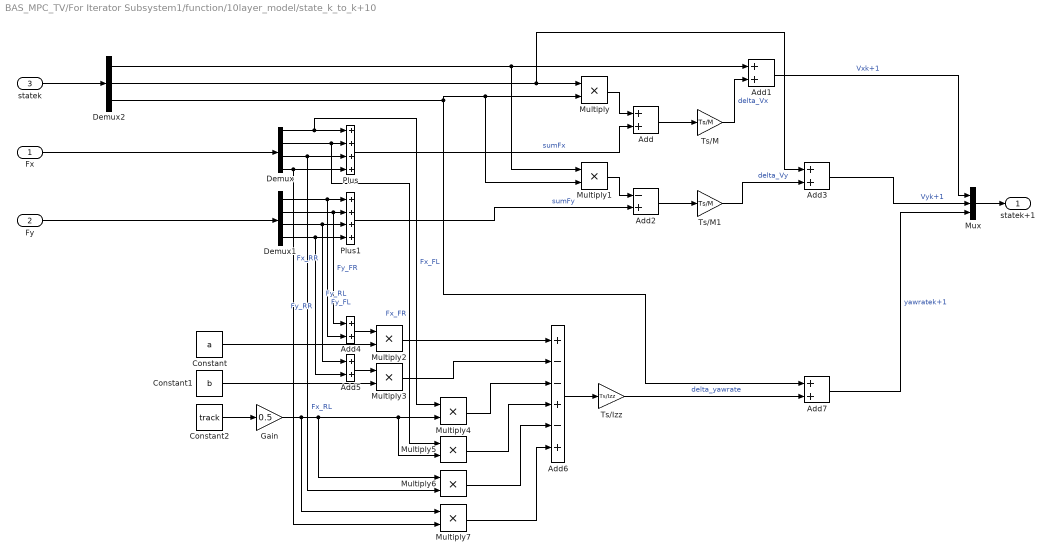
== system BAS_MPC_TV/For Iterator Subsystem1/function/10layer_model/state_k_to_k+10 ==
  Fx : Inport
  Fy : Inport  Port=2
  statek : Inport  Port=3
  Add{,1,3..5,7} (6 alike) : Sum
  Add2 : Sum  Inputs=-+
  Add6 : Sum  Inputs=+--+-+
  Constant : Constant  Value=a
  Constant1 : Constant  Value=b
  Constant2 : Constant  Value=track
  Demux : Demux
  Demux1 : Demux
  Demux2 : Demux  Outputs=3
  Gain : Gain  Gain=0.5
  Multiply{,1..7} (8 alike) : Product
  Mux : Mux  Inputs=3
  Plus : Sum  Inputs=4
  Plus1 : Sum  Inputs=4
  Ts/Izz : Gain  Gain=Ts/Izz
  Ts/M : Gain  Gain=Ts/M
  Ts/M1 : Gain  Gain=Ts/M
  statek+1 : Outport
  wires:
  Demux2/2 -> Add3/1, Multiply/1
  Demux2/3 -> Multiply1/2, Multiply/2, Add7/1
  Multiply/1 -> Add/1
  Add/1 -> Ts/M/1
  Ts/M/1 -> Add1/2  "delta_Vx"
  Demux2/1 -> Add1/1, Multiply1/1
  Add1/1 -> Mux/1  "Vxk+1"
  Fx/1 -> Demux/1
  Demux/1 -> Multiply4/1, Plus/1  "Fx_FL"
  Demux/2 -> Multiply5/1, Plus/2  "Fx_FR"
  Demux/3 -> Multiply6/2, Plus/3  "Fx_RL"
  Demux/4 -> Plus/4, Multiply7/2  "Fx_RR"
  Plus/1 -> Add/2  "sumFx"
  Demux1/3 -> Add5/1, Plus1/3  "Fy_RL"
  Demux1/2 -> Add4/1, Plus1/2  "Fy_FR"
  Demux1/1 -> Add4/2, Plus1/1  "Fy_FL"
  Demux1/4 -> Add5/2, Plus1/4  "Fy_RR"
  Fy/1 -> Demux1/1
  Plus1/1 -> Add2/2  "sumFy"
  Multiply1/1 -> Add2/1
  Add2/1 -> Ts/M1/1
  Ts/M1/1 -> Add3/2  "delta_Vy"
  Add3/1 -> Mux/2  "Vyk+1"
  Add4/1 -> Multiply2/1
  Constant/1 -> Multiply2/2
  Multiply2/1 -> Add6/1
  Multiply3/1 -> Add6/2
  Constant1/1 -> Multiply3/2
  Add5/1 -> Multiply3/1
  Constant2/1 -> Gain/1
  Gain/1 -> Multiply7/1, Multiply4/2, Multiply5/2, Multiply6/1
  Multiply4/1 -> Add6/3
  Multiply5/1 -> Add6/4
  Multiply6/1 -> Add6/5
  Multiply7/1 -> Add6/6
  Add6/1 -> Ts/Izz/1
  Ts/Izz/1 -> Add7/2  "delta_yawrate"
  Add7/1 -> Mux/3  "yawratek+1"
  statek/1 -> Demux2/1
  Mux/1 -> statek+1/1

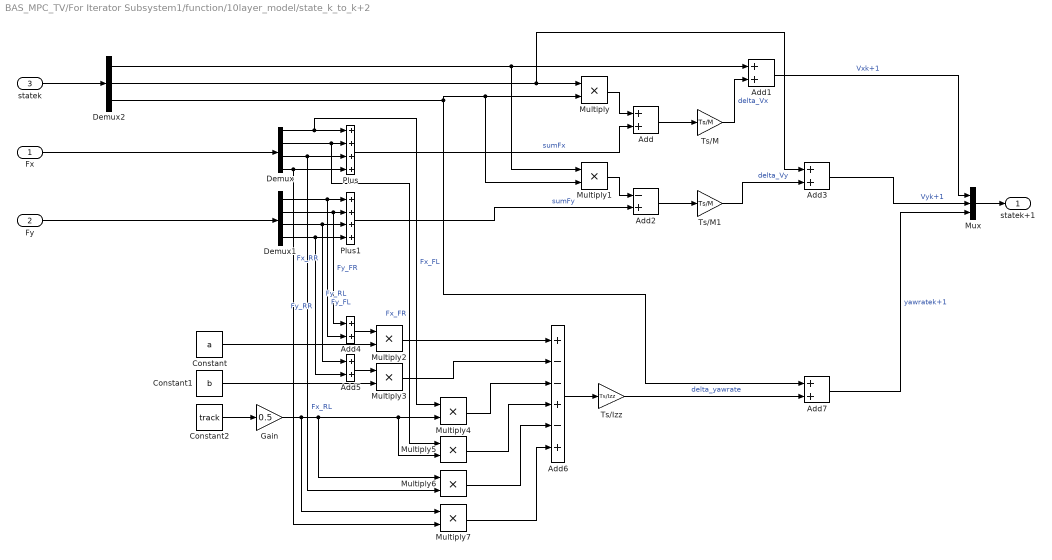
== system BAS_MPC_TV/For Iterator Subsystem1/function/10layer_model/state_k_to_k+2 ==
  Fx : Inport
  Fy : Inport  Port=2
  statek : Inport  Port=3
  Add{,1,3..5,7} (6 alike) : Sum
  Add2 : Sum  Inputs=-+
  Add6 : Sum  Inputs=+--+-+
  Constant : Constant  Value=a
  Constant1 : Constant  Value=b
  Constant2 : Constant  Value=track
  Demux : Demux
  Demux1 : Demux
  Demux2 : Demux  Outputs=3
  Gain : Gain  Gain=0.5
  Multiply{,1..7} (8 alike) : Product
  Mux : Mux  Inputs=3
  Plus : Sum  Inputs=4
  Plus1 : Sum  Inputs=4
  Ts/Izz : Gain  Gain=Ts/Izz
  Ts/M : Gain  Gain=Ts/M
  Ts/M1 : Gain  Gain=Ts/M
  statek+1 : Outport
  wires:
  Demux2/2 -> Add3/1, Multiply/1
  Demux2/3 -> Multiply1/2, Multiply/2, Add7/1
  Multiply/1 -> Add/1
  Add/1 -> Ts/M/1
  Ts/M/1 -> Add1/2  "delta_Vx"
  Demux2/1 -> Add1/1, Multiply1/1
  Add1/1 -> Mux/1  "Vxk+1"
  Fx/1 -> Demux/1
  Demux/1 -> Multiply4/1, Plus/1  "Fx_FL"
  Demux/2 -> Multiply5/1, Plus/2  "Fx_FR"
  Demux/3 -> Multiply6/2, Plus/3  "Fx_RL"
  Demux/4 -> Plus/4, Multiply7/2  "Fx_RR"
  Plus/1 -> Add/2  "sumFx"
  Demux1/3 -> Add5/1, Plus1/3  "Fy_RL"
  Demux1/2 -> Add4/1, Plus1/2  "Fy_FR"
  Demux1/1 -> Add4/2, Plus1/1  "Fy_FL"
  Demux1/4 -> Add5/2, Plus1/4  "Fy_RR"
  Fy/1 -> Demux1/1
  Plus1/1 -> Add2/2  "sumFy"
  Multiply1/1 -> Add2/1
  Add2/1 -> Ts/M1/1
  Ts/M1/1 -> Add3/2  "delta_Vy"
  Add3/1 -> Mux/2  "Vyk+1"
  Add4/1 -> Multiply2/1
  Constant/1 -> Multiply2/2
  Multiply2/1 -> Add6/1
  Multiply3/1 -> Add6/2
  Constant1/1 -> Multiply3/2
  Add5/1 -> Multiply3/1
  Constant2/1 -> Gain/1
  Gain/1 -> Multiply7/1, Multiply4/2, Multiply5/2, Multiply6/1
  Multiply4/1 -> Add6/3
  Multiply5/1 -> Add6/4
  Multiply6/1 -> Add6/5
  Multiply7/1 -> Add6/6
  Add6/1 -> Ts/Izz/1
  Ts/Izz/1 -> Add7/2  "delta_yawrate"
  Add7/1 -> Mux/3  "yawratek+1"
  statek/1 -> Demux2/1
  Mux/1 -> statek+1/1

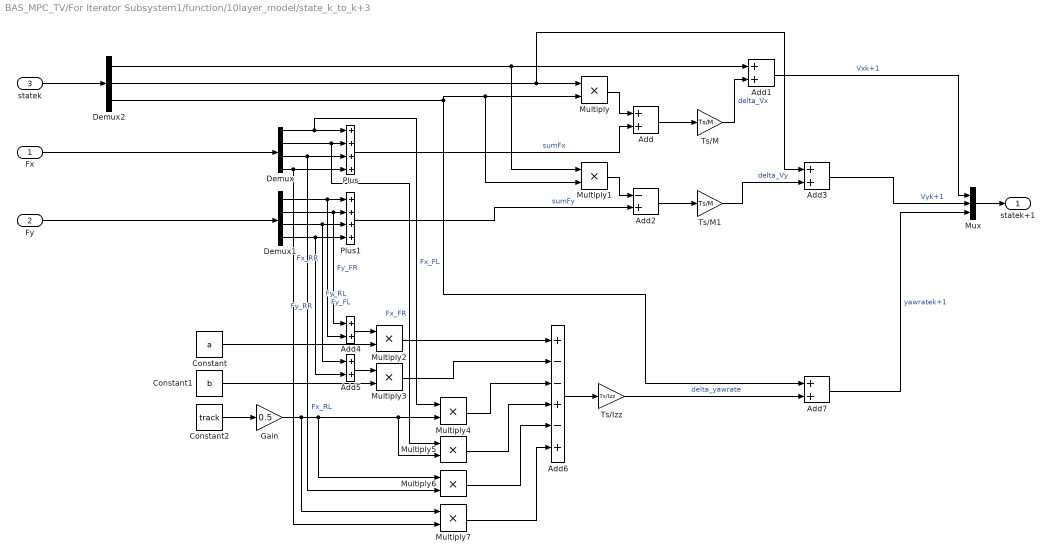
== system BAS_MPC_TV/For Iterator Subsystem1/function/10layer_model/state_k_to_k+3 ==
  Fx : Inport
  Fy : Inport  Port=2
  statek : Inport  Port=3
  Add{,1,3..5,7} (6 alike) : Sum
  Add2 : Sum  Inputs=-+
  Add6 : Sum  Inputs=+--+-+
  Constant : Constant  Value=a
  Constant1 : Constant  Value=b
  Constant2 : Constant  Value=track
  Demux : Demux
  Demux1 : Demux
  Demux2 : Demux  Outputs=3
  Gain : Gain  Gain=0.5
  Multiply{,1..7} (8 alike) : Product
  Mux : Mux  Inputs=3
  Plus : Sum  Inputs=4
  Plus1 : Sum  Inputs=4
  Ts/Izz : Gain  Gain=Ts/Izz
  Ts/M : Gain  Gain=Ts/M
  Ts/M1 : Gain  Gain=Ts/M
  statek+1 : Outport
  wires:
  Demux2/2 -> Add3/1, Multiply/1
  Demux2/3 -> Multiply1/2, Multiply/2, Add7/1
  Multiply/1 -> Add/1
  Add/1 -> Ts/M/1
  Ts/M/1 -> Add1/2  "delta_Vx"
  Demux2/1 -> Add1/1, Multiply1/1
  Add1/1 -> Mux/1  "Vxk+1"
  Fx/1 -> Demux/1
  Demux/1 -> Multiply4/1, Plus/1  "Fx_FL"
  Demux/2 -> Multiply5/1, Plus/2  "Fx_FR"
  Demux/3 -> Multiply6/2, Plus/3  "Fx_RL"
  Demux/4 -> Plus/4, Multiply7/2  "Fx_RR"
  Plus/1 -> Add/2  "sumFx"
  Demux1/3 -> Add5/1, Plus1/3  "Fy_RL"
  Demux1/2 -> Add4/1, Plus1/2  "Fy_FR"
  Demux1/1 -> Add4/2, Plus1/1  "Fy_FL"
  Demux1/4 -> Add5/2, Plus1/4  "Fy_RR"
  Fy/1 -> Demux1/1
  Plus1/1 -> Add2/2  "sumFy"
  Multiply1/1 -> Add2/1
  Add2/1 -> Ts/M1/1
  Ts/M1/1 -> Add3/2  "delta_Vy"
  Add3/1 -> Mux/2  "Vyk+1"
  Add4/1 -> Multiply2/1
  Constant/1 -> Multiply2/2
  Multiply2/1 -> Add6/1
  Multiply3/1 -> Add6/2
  Constant1/1 -> Multiply3/2
  Add5/1 -> Multiply3/1
  Constant2/1 -> Gain/1
  Gain/1 -> Multiply7/1, Multiply4/2, Multiply5/2, Multiply6/1
  Multiply4/1 -> Add6/3
  Multiply5/1 -> Add6/4
  Multiply6/1 -> Add6/5
  Multiply7/1 -> Add6/6
  Add6/1 -> Ts/Izz/1
  Ts/Izz/1 -> Add7/2  "delta_yawrate"
  Add7/1 -> Mux/3  "yawratek+1"
  statek/1 -> Demux2/1
  Mux/1 -> statek+1/1

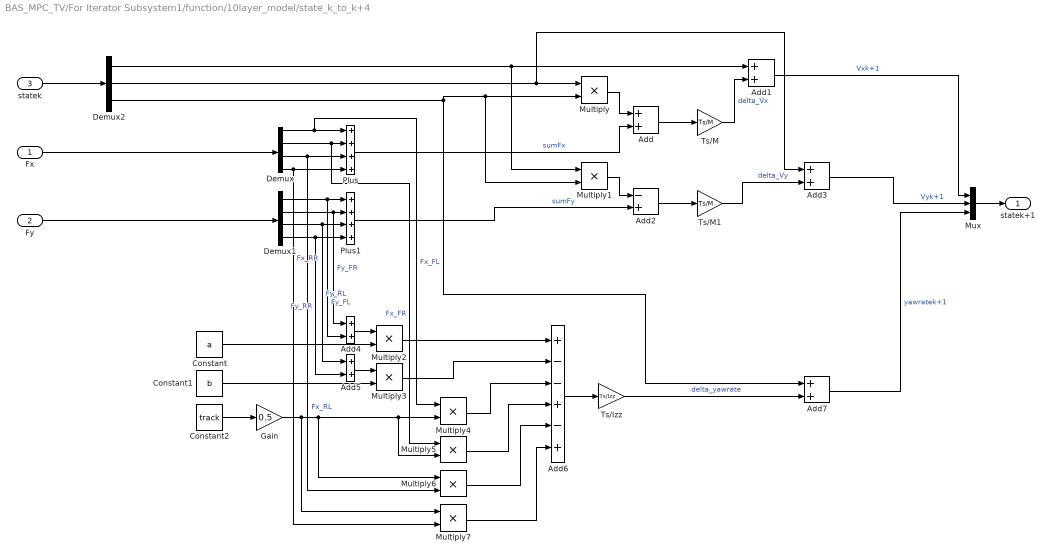
== system BAS_MPC_TV/For Iterator Subsystem1/function/10layer_model/state_k_to_k+4 ==
  Fx : Inport
  Fy : Inport  Port=2
  statek : Inport  Port=3
  Add{,1,3..5,7} (6 alike) : Sum
  Add2 : Sum  Inputs=-+
  Add6 : Sum  Inputs=+--+-+
  Constant : Constant  Value=a
  Constant1 : Constant  Value=b
  Constant2 : Constant  Value=track
  Demux : Demux
  Demux1 : Demux
  Demux2 : Demux  Outputs=3
  Gain : Gain  Gain=0.5
  Multiply{,1..7} (8 alike) : Product
  Mux : Mux  Inputs=3
  Plus : Sum  Inputs=4
  Plus1 : Sum  Inputs=4
  Ts/Izz : Gain  Gain=Ts/Izz
  Ts/M : Gain  Gain=Ts/M
  Ts/M1 : Gain  Gain=Ts/M
  statek+1 : Outport
  wires:
  Demux2/2 -> Add3/1, Multiply/1
  Demux2/3 -> Multiply1/2, Multiply/2, Add7/1
  Multiply/1 -> Add/1
  Add/1 -> Ts/M/1
  Ts/M/1 -> Add1/2  "delta_Vx"
  Demux2/1 -> Add1/1, Multiply1/1
  Add1/1 -> Mux/1  "Vxk+1"
  Fx/1 -> Demux/1
  Demux/1 -> Multiply4/1, Plus/1  "Fx_FL"
  Demux/2 -> Multiply5/1, Plus/2  "Fx_FR"
  Demux/3 -> Multiply6/2, Plus/3  "Fx_RL"
  Demux/4 -> Plus/4, Multiply7/2  "Fx_RR"
  Plus/1 -> Add/2  "sumFx"
  Demux1/3 -> Add5/1, Plus1/3  "Fy_RL"
  Demux1/2 -> Add4/1, Plus1/2  "Fy_FR"
  Demux1/1 -> Add4/2, Plus1/1  "Fy_FL"
  Demux1/4 -> Add5/2, Plus1/4  "Fy_RR"
  Fy/1 -> Demux1/1
  Plus1/1 -> Add2/2  "sumFy"
  Multiply1/1 -> Add2/1
  Add2/1 -> Ts/M1/1
  Ts/M1/1 -> Add3/2  "delta_Vy"
  Add3/1 -> Mux/2  "Vyk+1"
  Add4/1 -> Multiply2/1
  Constant/1 -> Multiply2/2
  Multiply2/1 -> Add6/1
  Multiply3/1 -> Add6/2
  Constant1/1 -> Multiply3/2
  Add5/1 -> Multiply3/1
  Constant2/1 -> Gain/1
  Gain/1 -> Multiply7/1, Multiply4/2, Multiply5/2, Multiply6/1
  Multiply4/1 -> Add6/3
  Multiply5/1 -> Add6/4
  Multiply6/1 -> Add6/5
  Multiply7/1 -> Add6/6
  Add6/1 -> Ts/Izz/1
  Ts/Izz/1 -> Add7/2  "delta_yawrate"
  Add7/1 -> Mux/3  "yawratek+1"
  statek/1 -> Demux2/1
  Mux/1 -> statek+1/1

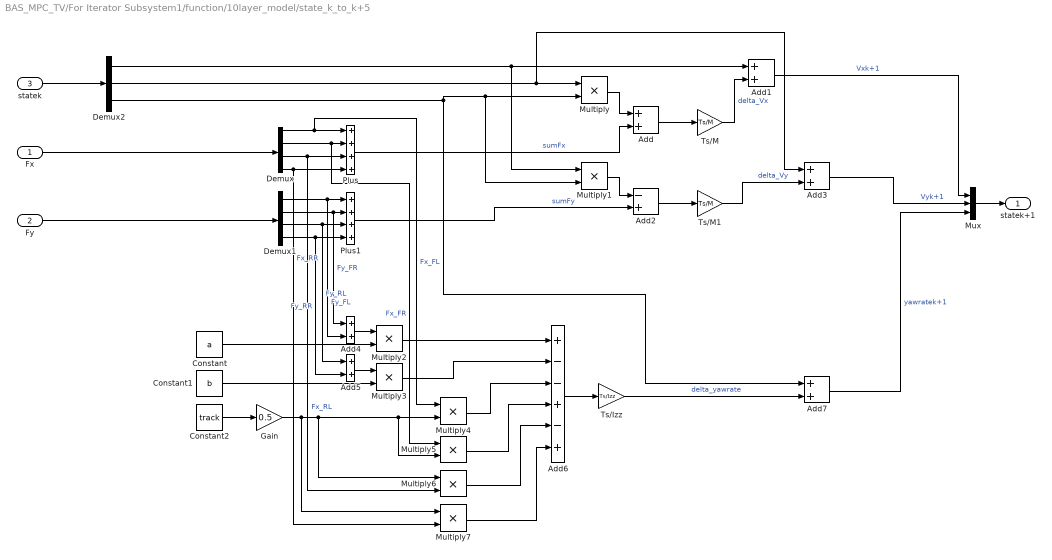
== system BAS_MPC_TV/For Iterator Subsystem1/function/10layer_model/state_k_to_k+5 ==
  Fx : Inport
  Fy : Inport  Port=2
  statek : Inport  Port=3
  Add{,1,3..5,7} (6 alike) : Sum
  Add2 : Sum  Inputs=-+
  Add6 : Sum  Inputs=+--+-+
  Constant : Constant  Value=a
  Constant1 : Constant  Value=b
  Constant2 : Constant  Value=track
  Demux : Demux
  Demux1 : Demux
  Demux2 : Demux  Outputs=3
  Gain : Gain  Gain=0.5
  Multiply{,1..7} (8 alike) : Product
  Mux : Mux  Inputs=3
  Plus : Sum  Inputs=4
  Plus1 : Sum  Inputs=4
  Ts/Izz : Gain  Gain=Ts/Izz
  Ts/M : Gain  Gain=Ts/M
  Ts/M1 : Gain  Gain=Ts/M
  statek+1 : Outport
  wires:
  Demux2/2 -> Add3/1, Multiply/1
  Demux2/3 -> Multiply1/2, Multiply/2, Add7/1
  Multiply/1 -> Add/1
  Add/1 -> Ts/M/1
  Ts/M/1 -> Add1/2  "delta_Vx"
  Demux2/1 -> Add1/1, Multiply1/1
  Add1/1 -> Mux/1  "Vxk+1"
  Fx/1 -> Demux/1
  Demux/1 -> Multiply4/1, Plus/1  "Fx_FL"
  Demux/2 -> Multiply5/1, Plus/2  "Fx_FR"
  Demux/3 -> Multiply6/2, Plus/3  "Fx_RL"
  Demux/4 -> Plus/4, Multiply7/2  "Fx_RR"
  Plus/1 -> Add/2  "sumFx"
  Demux1/3 -> Add5/1, Plus1/3  "Fy_RL"
  Demux1/2 -> Add4/1, Plus1/2  "Fy_FR"
  Demux1/1 -> Add4/2, Plus1/1  "Fy_FL"
  Demux1/4 -> Add5/2, Plus1/4  "Fy_RR"
  Fy/1 -> Demux1/1
  Plus1/1 -> Add2/2  "sumFy"
  Multiply1/1 -> Add2/1
  Add2/1 -> Ts/M1/1
  Ts/M1/1 -> Add3/2  "delta_Vy"
  Add3/1 -> Mux/2  "Vyk+1"
  Add4/1 -> Multiply2/1
  Constant/1 -> Multiply2/2
  Multiply2/1 -> Add6/1
  Multiply3/1 -> Add6/2
  Constant1/1 -> Multiply3/2
  Add5/1 -> Multiply3/1
  Constant2/1 -> Gain/1
  Gain/1 -> Multiply7/1, Multiply4/2, Multiply5/2, Multiply6/1
  Multiply4/1 -> Add6/3
  Multiply5/1 -> Add6/4
  Multiply6/1 -> Add6/5
  Multiply7/1 -> Add6/6
  Add6/1 -> Ts/Izz/1
  Ts/Izz/1 -> Add7/2  "delta_yawrate"
  Add7/1 -> Mux/3  "yawratek+1"
  statek/1 -> Demux2/1
  Mux/1 -> statek+1/1

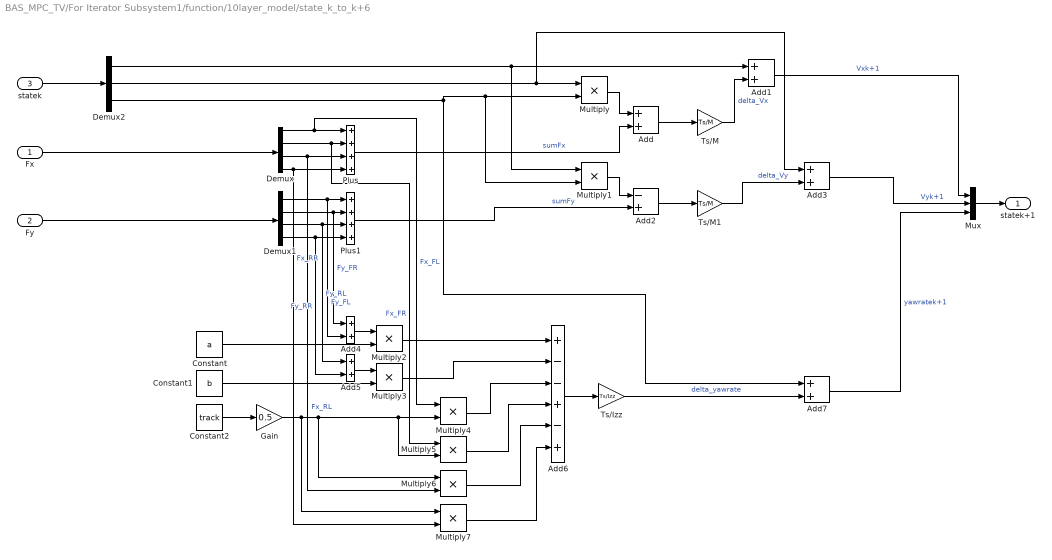
== system BAS_MPC_TV/For Iterator Subsystem1/function/10layer_model/state_k_to_k+6 ==
  Fx : Inport
  Fy : Inport  Port=2
  statek : Inport  Port=3
  Add{,1,3..5,7} (6 alike) : Sum
  Add2 : Sum  Inputs=-+
  Add6 : Sum  Inputs=+--+-+
  Constant : Constant  Value=a
  Constant1 : Constant  Value=b
  Constant2 : Constant  Value=track
  Demux : Demux
  Demux1 : Demux
  Demux2 : Demux  Outputs=3
  Gain : Gain  Gain=0.5
  Multiply{,1..7} (8 alike) : Product
  Mux : Mux  Inputs=3
  Plus : Sum  Inputs=4
  Plus1 : Sum  Inputs=4
  Ts/Izz : Gain  Gain=Ts/Izz
  Ts/M : Gain  Gain=Ts/M
  Ts/M1 : Gain  Gain=Ts/M
  statek+1 : Outport
  wires:
  Demux2/2 -> Add3/1, Multiply/1
  Demux2/3 -> Multiply1/2, Multiply/2, Add7/1
  Multiply/1 -> Add/1
  Add/1 -> Ts/M/1
  Ts/M/1 -> Add1/2  "delta_Vx"
  Demux2/1 -> Add1/1, Multiply1/1
  Add1/1 -> Mux/1  "Vxk+1"
  Fx/1 -> Demux/1
  Demux/1 -> Multiply4/1, Plus/1  "Fx_FL"
  Demux/2 -> Multiply5/1, Plus/2  "Fx_FR"
  Demux/3 -> Multiply6/2, Plus/3  "Fx_RL"
  Demux/4 -> Plus/4, Multiply7/2  "Fx_RR"
  Plus/1 -> Add/2  "sumFx"
  Demux1/3 -> Add5/1, Plus1/3  "Fy_RL"
  Demux1/2 -> Add4/1, Plus1/2  "Fy_FR"
  Demux1/1 -> Add4/2, Plus1/1  "Fy_FL"
  Demux1/4 -> Add5/2, Plus1/4  "Fy_RR"
  Fy/1 -> Demux1/1
  Plus1/1 -> Add2/2  "sumFy"
  Multiply1/1 -> Add2/1
  Add2/1 -> Ts/M1/1
  Ts/M1/1 -> Add3/2  "delta_Vy"
  Add3/1 -> Mux/2  "Vyk+1"
  Add4/1 -> Multiply2/1
  Constant/1 -> Multiply2/2
  Multiply2/1 -> Add6/1
  Multiply3/1 -> Add6/2
  Constant1/1 -> Multiply3/2
  Add5/1 -> Multiply3/1
  Constant2/1 -> Gain/1
  Gain/1 -> Multiply7/1, Multiply4/2, Multiply5/2, Multiply6/1
  Multiply4/1 -> Add6/3
  Multiply5/1 -> Add6/4
  Multiply6/1 -> Add6/5
  Multiply7/1 -> Add6/6
  Add6/1 -> Ts/Izz/1
  Ts/Izz/1 -> Add7/2  "delta_yawrate"
  Add7/1 -> Mux/3  "yawratek+1"
  statek/1 -> Demux2/1
  Mux/1 -> statek+1/1

== system BAS_MPC_TV/For Iterator Subsystem1/function/10layer_model/state_k_to_k+7 ==
  Fx : Inport
  Fy : Inport  Port=2
  statek : Inport  Port=3
  Add{,1,3..5,7} (6 alike) : Sum
  Add2 : Sum  Inputs=-+
  Add6 : Sum  Inputs=+--+-+
  Constant : Constant  Value=a
  Constant1 : Constant  Value=b
  Constant2 : Constant  Value=track
  Demux : Demux
  Demux1 : Demux
  Demux2 : Demux  Outputs=3
  Gain : Gain  Gain=0.5
  Multiply{,1..7} (8 alike) : Product
  Mux : Mux  Inputs=3
  Plus : Sum  Inputs=4
  Plus1 : Sum  Inputs=4
  Ts/Izz : Gain  Gain=Ts/Izz
  Ts/M : Gain  Gain=Ts/M
  Ts/M1 : Gain  Gain=Ts/M
  statek+1 : Outport
  wires:
  Demux2/2 -> Add3/1, Multiply/1
  Demux2/3 -> Multiply1/2, Multiply/2, Add7/1
  Multiply/1 -> Add/1
  Add/1 -> Ts/M/1
  Ts/M/1 -> Add1/2  "delta_Vx"
  Demux2/1 -> Add1/1, Multiply1/1
  Add1/1 -> Mux/1  "Vxk+1"
  Fx/1 -> Demux/1
  Demux/1 -> Multiply4/1, Plus/1  "Fx_FL"
  Demux/2 -> Multiply5/1, Plus/2  "Fx_FR"
  Demux/3 -> Multiply6/2, Plus/3  "Fx_RL"
  Demux/4 -> Plus/4, Multiply7/2  "Fx_RR"
  Plus/1 -> Add/2  "sumFx"
  Demux1/3 -> Add5/1, Plus1/3  "Fy_RL"
  Demux1/2 -> Add4/1, Plus1/2  "Fy_FR"
  Demux1/1 -> Add4/2, Plus1/1  "Fy_FL"
  Demux1/4 -> Add5/2, Plus1/4  "Fy_RR"
  Fy/1 -> Demux1/1
  Plus1/1 -> Add2/2  "sumFy"
  Multiply1/1 -> Add2/1
  Add2/1 -> Ts/M1/1
  Ts/M1/1 -> Add3/2  "delta_Vy"
  Add3/1 -> Mux/2  "Vyk+1"
  Add4/1 -> Multiply2/1
  Constant/1 -> Multiply2/2
  Multiply2/1 -> Add6/1
  Multiply3/1 -> Add6/2
  Constant1/1 -> Multiply3/2
  Add5/1 -> Multiply3/1
  Constant2/1 -> Gain/1
  Gain/1 -> Multiply7/1, Multiply4/2, Multiply5/2, Multiply6/1
  Multiply4/1 -> Add6/3
  Multiply5/1 -> Add6/4
  Multiply6/1 -> Add6/5
  Multiply7/1 -> Add6/6
  Add6/1 -> Ts/Izz/1
  Ts/Izz/1 -> Add7/2  "delta_yawrate"
  Add7/1 -> Mux/3  "yawratek+1"
  statek/1 -> Demux2/1
  Mux/1 -> statek+1/1

== system BAS_MPC_TV/For Iterator Subsystem1/function/10layer_model/state_k_to_k+8 ==
  Fx : Inport
  Fy : Inport  Port=2
  statek : Inport  Port=3
  Add{,1,3..5,7} (6 alike) : Sum
  Add2 : Sum  Inputs=-+
  Add6 : Sum  Inputs=+--+-+
  Constant : Constant  Value=a
  Constant1 : Constant  Value=b
  Constant2 : Constant  Value=track
  Demux : Demux
  Demux1 : Demux
  Demux2 : Demux  Outputs=3
  Gain : Gain  Gain=0.5
  Multiply{,1..7} (8 alike) : Product
  Mux : Mux  Inputs=3
  Plus : Sum  Inputs=4
  Plus1 : Sum  Inputs=4
  Ts/Izz : Gain  Gain=Ts/Izz
  Ts/M : Gain  Gain=Ts/M
  Ts/M1 : Gain  Gain=Ts/M
  statek+1 : Outport
  wires:
  Demux2/2 -> Add3/1, Multiply/1
  Demux2/3 -> Multiply1/2, Multiply/2, Add7/1
  Multiply/1 -> Add/1
  Add/1 -> Ts/M/1
  Ts/M/1 -> Add1/2  "delta_Vx"
  Demux2/1 -> Add1/1, Multiply1/1
  Add1/1 -> Mux/1  "Vxk+1"
  Fx/1 -> Demux/1
  Demux/1 -> Multiply4/1, Plus/1  "Fx_FL"
  Demux/2 -> Multiply5/1, Plus/2  "Fx_FR"
  Demux/3 -> Multiply6/2, Plus/3  "Fx_RL"
  Demux/4 -> Plus/4, Multiply7/2  "Fx_RR"
  Plus/1 -> Add/2  "sumFx"
  Demux1/3 -> Add5/1, Plus1/3  "Fy_RL"
  Demux1/2 -> Add4/1, Plus1/2  "Fy_FR"
  Demux1/1 -> Add4/2, Plus1/1  "Fy_FL"
  Demux1/4 -> Add5/2, Plus1/4  "Fy_RR"
  Fy/1 -> Demux1/1
  Plus1/1 -> Add2/2  "sumFy"
  Multiply1/1 -> Add2/1
  Add2/1 -> Ts/M1/1
  Ts/M1/1 -> Add3/2  "delta_Vy"
  Add3/1 -> Mux/2  "Vyk+1"
  Add4/1 -> Multiply2/1
  Constant/1 -> Multiply2/2
  Multiply2/1 -> Add6/1
  Multiply3/1 -> Add6/2
  Constant1/1 -> Multiply3/2
  Add5/1 -> Multiply3/1
  Constant2/1 -> Gain/1
  Gain/1 -> Multiply7/1, Multiply4/2, Multiply5/2, Multiply6/1
  Multiply4/1 -> Add6/3
  Multiply5/1 -> Add6/4
  Multiply6/1 -> Add6/5
  Multiply7/1 -> Add6/6
  Add6/1 -> Ts/Izz/1
  Ts/Izz/1 -> Add7/2  "delta_yawrate"
  Add7/1 -> Mux/3  "yawratek+1"
  statek/1 -> Demux2/1
  Mux/1 -> statek+1/1

== system BAS_MPC_TV/For Iterator Subsystem1/function/10layer_model/state_k_to_k+9 ==
  Fx : Inport
  Fy : Inport  Port=2
  statek : Inport  Port=3
  Add{,1,3..5,7} (6 alike) : Sum
  Add2 : Sum  Inputs=-+
  Add6 : Sum  Inputs=+--+-+
  Constant : Constant  Value=a
  Constant1 : Constant  Value=b
  Constant2 : Constant  Value=track
  Demux : Demux
  Demux1 : Demux
  Demux2 : Demux  Outputs=3
  Gain : Gain  Gain=0.5
  Multiply{,1..7} (8 alike) : Product
  Mux : Mux  Inputs=3
  Plus : Sum  Inputs=4
  Plus1 : Sum  Inputs=4
  Ts/Izz : Gain  Gain=Ts/Izz
  Ts/M : Gain  Gain=Ts/M
  Ts/M1 : Gain  Gain=Ts/M
  statek+1 : Outport
  wires:
  Demux2/2 -> Add3/1, Multiply/1
  Demux2/3 -> Multiply1/2, Multiply/2, Add7/1
  Multiply/1 -> Add/1
  Add/1 -> Ts/M/1
  Ts/M/1 -> Add1/2  "delta_Vx"
  Demux2/1 -> Add1/1, Multiply1/1
  Add1/1 -> Mux/1  "Vxk+1"
  Fx/1 -> Demux/1
  Demux/1 -> Multiply4/1, Plus/1  "Fx_FL"
  Demux/2 -> Multiply5/1, Plus/2  "Fx_FR"
  Demux/3 -> Multiply6/2, Plus/3  "Fx_RL"
  Demux/4 -> Plus/4, Multiply7/2  "Fx_RR"
  Plus/1 -> Add/2  "sumFx"
  Demux1/3 -> Add5/1, Plus1/3  "Fy_RL"
  Demux1/2 -> Add4/1, Plus1/2  "Fy_FR"
  Demux1/1 -> Add4/2, Plus1/1  "Fy_FL"
  Demux1/4 -> Add5/2, Plus1/4  "Fy_RR"
  Fy/1 -> Demux1/1
  Plus1/1 -> Add2/2  "sumFy"
  Multiply1/1 -> Add2/1
  Add2/1 -> Ts/M1/1
  Ts/M1/1 -> Add3/2  "delta_Vy"
  Add3/1 -> Mux/2  "Vyk+1"
  Add4/1 -> Multiply2/1
  Constant/1 -> Multiply2/2
  Multiply2/1 -> Add6/1
  Multiply3/1 -> Add6/2
  Constant1/1 -> Multiply3/2
  Add5/1 -> Multiply3/1
  Constant2/1 -> Gain/1
  Gain/1 -> Multiply7/1, Multiply4/2, Multiply5/2, Multiply6/1
  Multiply4/1 -> Add6/3
  Multiply5/1 -> Add6/4
  Multiply6/1 -> Add6/5
  Multiply7/1 -> Add6/6
  Add6/1 -> Ts/Izz/1
  Ts/Izz/1 -> Add7/2  "delta_yawrate"
  Add7/1 -> Mux/3  "yawratek+1"
  statek/1 -> Demux2/1
  Mux/1 -> statek+1/1

== system BAS_MPC_TV/For Iterator Subsystem1/function1/10layer_model/state_k_to_k+1 ==
  Fx : Inport
  Fy : Inport  Port=2
  statek : Inport  Port=3
  Add{,1,3..5,7} (6 alike) : Sum
  Add2 : Sum  Inputs=-+
  Add6 : Sum  Inputs=+--+-+
  Constant : Constant  Value=a
  Constant1 : Constant  Value=b
  Constant2 : Constant  Value=track
  Demux : Demux
  Demux1 : Demux
  Demux2 : Demux  Outputs=3
  Gain : Gain  Gain=0.5
  Multiply{,1..7} (8 alike) : Product
  Mux : Mux  Inputs=3
  Plus : Sum  Inputs=4
  Plus1 : Sum  Inputs=4
  Ts/Izz : Gain  Gain=Ts/Izz
  Ts/M : Gain  Gain=Ts/M
  Ts/M1 : Gain  Gain=Ts/M
  statek+1 : Outport
  wires:
  Demux2/2 -> Add3/1, Multiply/1
  Demux2/3 -> Multiply1/2, Multiply/2, Add7/1
  Multiply/1 -> Add/1
  Add/1 -> Ts/M/1
  Ts/M/1 -> Add1/2  "delta_Vx"
  Demux2/1 -> Add1/1, Multiply1/1
  Add1/1 -> Mux/1  "Vxk+1"
  Fx/1 -> Demux/1
  Demux/1 -> Multiply4/1, Plus/1  "Fx_FL"
  Demux/2 -> Multiply5/1, Plus/2  "Fx_FR"
  Demux/3 -> Multiply6/2, Plus/3  "Fx_RL"
  Demux/4 -> Plus/4, Multiply7/2  "Fx_RR"
  Plus/1 -> Add/2  "sumFx"
  Demux1/3 -> Add5/1, Plus1/3  "Fy_RL"
  Demux1/2 -> Add4/1, Plus1/2  "Fy_FR"
  Demux1/1 -> Add4/2, Plus1/1  "Fy_FL"
  Demux1/4 -> Add5/2, Plus1/4  "Fy_RR"
  Fy/1 -> Demux1/1
  Plus1/1 -> Add2/2  "sumFy"
  Multiply1/1 -> Add2/1
  Add2/1 -> Ts/M1/1
  Ts/M1/1 -> Add3/2  "delta_Vy"
  Add3/1 -> Mux/2  "Vyk+1"
  Add4/1 -> Multiply2/1
  Constant/1 -> Multiply2/2
  Multiply2/1 -> Add6/1
  Multiply3/1 -> Add6/2
  Constant1/1 -> Multiply3/2
  Add5/1 -> Multiply3/1
  Constant2/1 -> Gain/1
  Gain/1 -> Multiply7/1, Multiply4/2, Multiply5/2, Multiply6/1
  Multiply4/1 -> Add6/3
  Multiply5/1 -> Add6/4
  Multiply6/1 -> Add6/5
  Multiply7/1 -> Add6/6
  Add6/1 -> Ts/Izz/1
  Ts/Izz/1 -> Add7/2  "delta_yawrate"
  Add7/1 -> Mux/3  "yawratek+1"
  statek/1 -> Demux2/1
  Mux/1 -> statek+1/1
